simulink model "exportTest"  (Simulink 7.8)
settings: Solver=ode45  StartTime=0.0  StopTime=10.0  RelTol=1e-3
settings Model: Creator=trommsdorff  LastModifiedBy=trommsdorff

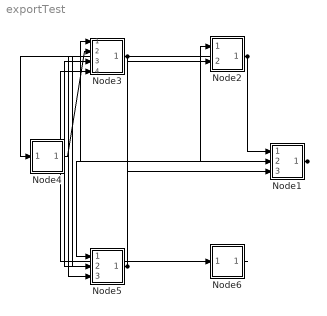
== system exportTest ==
  Node1 : Subsystem
  Node2 : Subsystem
  Node3 : Subsystem
  Node4 : Subsystem
  Node5 : Subsystem
  Node6 : Subsystem
  wires:
  Node1/1(Out1) -> Node2/1(In1), Node3/1(In1), Node5/1(In1)
  Node2/1(Out1) -> Node1/1(In2), Node5/2(In2)
  Node3/1(Out1) -> Node1/2(In3), Node4/1(In3), Node5/3(In3), Node6/1(In3)
  Node4/1(Out1) -> Node3/2(In4)
  Node5/1(Out1) -> Node1/3(In5), Node2/2(In5), Node3/3(In5)
  Node6/1(Out1) -> Node3/4(In6)

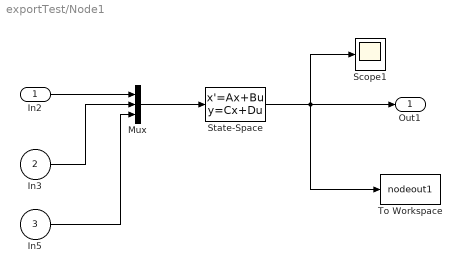
== system exportTest/Node1 ==
  In2 : Inport
  In3 : Inport  Port=2
  In5 : Inport  Port=3
  Mux : Mux  Inputs=3
  Scope1 : Scope
      settings: TimeRange=0.5847953216374258  YMin=-0.1657458563535892  YMax=1.21546961325967
  State-Space : StateSpace  A=[0 -1;-1 0]  B="[0.33333     0.33333     0.33333;0.33333     0.33333     0.33333]"  C=randn(1,2)  D="[0.33333     0.33333     0.33333]"  X0=randn(2,1)
  To Workspace : ToWorkspace  VariableName=nodeout1  SampleTime=-1  SaveFormat=Structure With Time
  Out1 : Outport
  wires:
  In5/1 -> Mux/3
  In3/1 -> Mux/2
  Mux/1 -> State-Space/1
  State-Space/1 -> Scope1/1, To Workspace/1, Out1/1
  In2/1 -> Mux/1

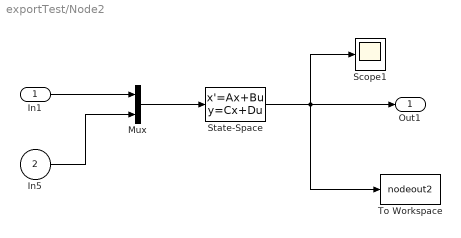
== system exportTest/Node2 ==
  In1 : Inport
  In5 : Inport  Port=2
  Mux : Mux  Inputs=2
  Scope1 : Scope
      settings: TimeRange=0.5847953216374258  YMin=-0.1657458563535892  YMax=1.21546961325967
  State-Space : StateSpace  A=[0 -1;-1 0]  B="[0.5         0.5;0.5         0.5]"  C=randn(1,2)  D="[0.5         0.5]"  X0=randn(2,1)
  To Workspace : ToWorkspace  VariableName=nodeout2  SampleTime=-1  SaveFormat=Structure With Time
  Out1 : Outport
  wires:
  In5/1 -> Mux/2
  Mux/1 -> State-Space/1
  State-Space/1 -> Scope1/1, To Workspace/1, Out1/1
  In1/1 -> Mux/1

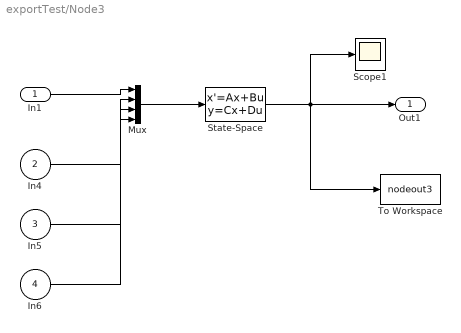
== system exportTest/Node3 ==
  In1 : Inport
  In4 : Inport  Port=2
  In5 : Inport  Port=3
  In6 : Inport  Port=4
  Mux : Mux
  Scope1 : Scope
      settings: TimeRange=0.5847953216374258  YMin=-0.1657458563535892  YMax=1.21546961325967
  State-Space : StateSpace  A=[0 -1;-1 0]  B="[0.25        0.25        0.25        0.25;0.25        0.25        0.25        0.25]"  C=randn(1,2)  D="[0.25        0.25        0.25        0.25]"  X0=randn(2,1)
  To Workspace : ToWorkspace  VariableName=nodeout3  SampleTime=-1  SaveFormat=Structure With Time
  Out1 : Outport
  wires:
  In6/1 -> Mux/4
  In5/1 -> Mux/3
  In4/1 -> Mux/2
  Mux/1 -> State-Space/1
  State-Space/1 -> Scope1/1, To Workspace/1, Out1/1
  In1/1 -> Mux/1

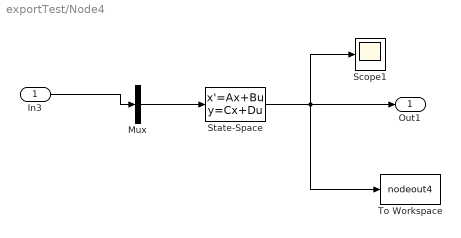
== system exportTest/Node4 ==
  In3 : Inport
  Mux : Mux  Inputs=1
  Scope1 : Scope
      settings: TimeRange=0.5847953216374258  YMin=-0.1657458563535892  YMax=1.21546961325967
  State-Space : StateSpace  A=[0 -1;-1 0]  B=randn(2,1)  C=randn(1,2)  D=zeros(1)  X0=randn(2,1)
  To Workspace : ToWorkspace  VariableName=nodeout4  SampleTime=-1  SaveFormat=Structure With Time
  Out1 : Outport
  wires:
  Mux/1 -> State-Space/1
  State-Space/1 -> Scope1/1, To Workspace/1, Out1/1
  In3/1 -> Mux/1

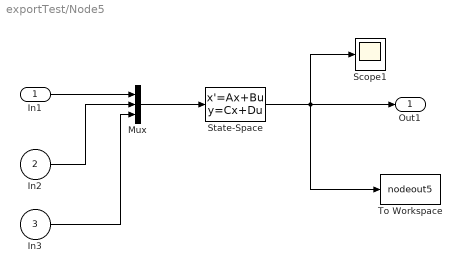
== system exportTest/Node5 ==
  In1 : Inport
  In2 : Inport  Port=2
  In3 : Inport  Port=3
  Mux : Mux  Inputs=3
  Scope1 : Scope
      settings: TimeRange=0.5847953216374258  YMin=-0.1657458563535892  YMax=1.21546961325967
  State-Space : StateSpace  A=[0 -1;-1 0]  B="[0.33333     0.33333     0.33333;0.33333     0.33333     0.33333]"  C=randn(1,2)  D="[0.33333     0.33333     0.33333]"  X0=randn(2,1)
  To Workspace : ToWorkspace  VariableName=nodeout5  SampleTime=-1  SaveFormat=Structure With Time
  Out1 : Outport
  wires:
  In3/1 -> Mux/3
  In2/1 -> Mux/2
  Mux/1 -> State-Space/1
  State-Space/1 -> Scope1/1, To Workspace/1, Out1/1
  In1/1 -> Mux/1

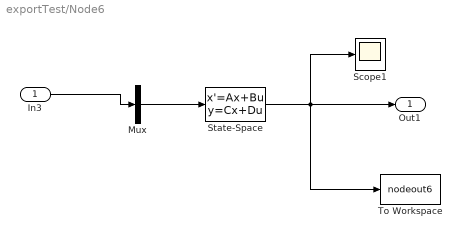
== system exportTest/Node6 ==
  In3 : Inport
  Mux : Mux  Inputs=1
  Scope1 : Scope
      settings: TimeRange=0.5847953216374258  YMin=-0.1657458563535892  YMax=1.21546961325967
  State-Space : StateSpace  A=[0 -1;-1 0]  B=randn(2,1)  C=randn(1,2)  D=zeros(1)  X0=randn(2,1)
  To Workspace : ToWorkspace  VariableName=nodeout6  SampleTime=-1  SaveFormat=Structure With Time
  Out1 : Outport
  wires:
  Mux/1 -> State-Space/1
  State-Space/1 -> Scope1/1, To Workspace/1, Out1/1
  In3/1 -> Mux/1
